simulink model "Monitor"  (R2022b)
settings: Solver=ode1  StartTime=0.0  StopTime=0.2  FixedStep=ctrlConst.TsSwitch  MaxStep=1e-6  RelTol=1e-3  EnableMultiTasking=on
PreLoadFcn:
  | %rtwdemo_pmsmfoc_data
StartFcn:
  | %clear executionProfile
StopFcn:
  | %try
  | %  AddExecutionProfileToDataInspector();
  | %end
undefined symbols (not defined in the file or in its folder): dataIphaOfsRawMon_C, facAdc2iPhMon_C, facAdc2uDclnkMon_C, KiRslvMonPI_C, KpRslvMonPI_C, Ld, Lq, Rss, SC_pMon_P, SC_PsiMon_P, tauTrqMonLv2_C, tauUdcPT1Mon_C, trqASCThdMonLv2_C, trqCmpThdMonLv2_C, Ts_10ms, Ts_1ms, Tsw
libraries: MathLib x14, IOLib x1, simulink x1
(part 2 of 2)

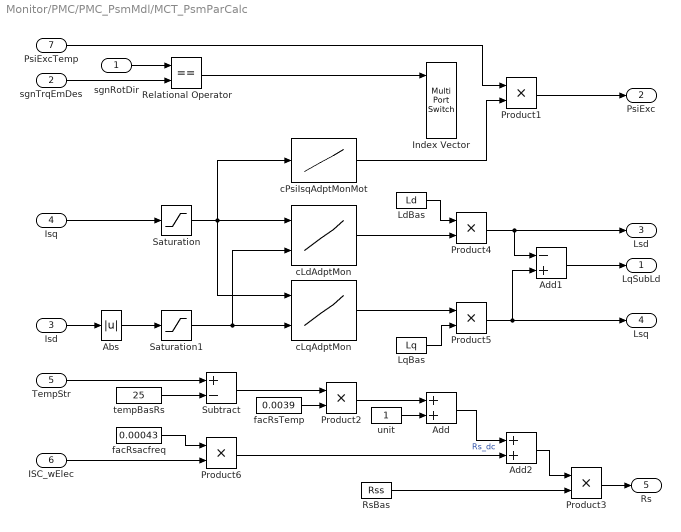
== system Monitor/PMC/PMC_PsmMdl/MCT_PsmParCalc ==
  sgnRotDir : Inport
  sgnTrqEmDes : Inport  Port=2
  Isd : Inport  Port=3
  Isq : Inport  Port=4
  TempStr : Inport  Port=5
  ISC_wElec : Inport  Port=6
  PsiExcTemp : Inport  Port=7
  Abs : Abs  SaturateOnIntegerOverflow=off
  Add : Sum  OutDataTypeStr=Inherit: Same as first input
  Add1 : Sum  Inputs=-+
  Add2 : Sum  OutDataTypeStr=Inherit: Same as first input
  Index Vector : MultiPortSwitch  DataPortOrder=Zero-based contiguous  Inputs=2  zeroidx=on  SaturateOnIntegerOverflow=off  InputSameDT=off
  LdBas : Constant  Value=Ld  OutDataTypeStr=single  SampleTime=-1
  LqBas : Constant  Value=Lq  OutDataTypeStr=single  SampleTime=-1
  Product1 : Product  OutDataTypeStr=single  RndMeth=Zero
  Product2 : Product  RndMeth=Zero
  Product3 : Product  RndMeth=Zero
  Product4 : Product  RndMeth=Zero  OutDataTypeStr=Inherit: Same as first input
  Product5 : Product  OutDataTypeStr=single  RndMeth=Zero
  Product6 : Product  RndMeth=Zero
  Relational Operator : RelationalOperator  Operator===  OutDataTypeStr=boolean  InputSameDT=off
  RsBas : Constant  Value=Rss  OutDataTypeStr=single  SampleTime=-1
  Saturation : Saturate  UpperLimit=450  LowerLimit=-450
  Saturation1 : Saturate  UpperLimit=450  LowerLimit=0
  Subtract : Sum  Inputs=+-
  cLdAdptMon : Lookup_n-D  DataSpecification=Lookup table object  LookupTableObject=cLdAdptMon_T  BreakpointsForDimension1=|  BreakpointsForDimension2=|  BeginIndexSearchUsingPreviousIndexResult=on  Table=|  ExtrapMethod=Clip  UseLastTableValue=on  InternalRulePriority=Speed  OutDataTypeStr=Inherit: Inherit from 'Table data'  InputSameDT=off
      BreakpointsForDimension1=|
      | [-530.4101839
      | -495.049505
      | -459.688826
      | -424.3281471
      | -388.9674682
      | -353.6067893
      | -318.2461103
      | -282.8854314
      | -247.5247525
      | -212.1640736
      | -176.8033946
      | -141.4427157
      | -106.0820368
      | -70.72135785
      | -35.36067893
      | 0
      | 35.36067893
      | 70.72135785
      | 106.0820368
      | 141.4427157
      | 176.8033946
      | 212.1640736
      | 247.5247525
      | 282.8854314
      | 318.2461103
      | 353.6067893
      | 388.9674682
      | 424.3281471
      | 459.688826
      | 495.049505
      | 530.4101839
      | ]
      BreakpointsForDimension2=|
      | [0	35.36067893	70.72135785	106.0820368	141.4427157	176.8033946	212.1640736	247.5247525	282.8854314	318.2461103	353.6067893	388.9674682	424.3281471	459.688826	495.049505	530.4101839
      | ]
      Table=|
      | [1	1	0.797297297	0.72972973	0.692567568	0.667567568	0.653153153	0.640926641	0.631756757	0.624624625	0.618918919	0.614742015	0.611486486	0.608731809	0.606177606	0.606177606
      | 1	1	0.797297297	0.72972973	0.692567568	0.667567568	0.653153153	0.640926641	0.631756757	0.624624625	0.618918919	0.614742015	0.611486486	0.608731809	0.606177606	0.606177606
      | 0.905405405	0.905405405	0.756756757	0.702702703	0.675675676	0.659459459	0.648648649	0.638996139	0.631756757	0.626126126	0.622972973	0.62002457	0.61768018	0.615800416	0.613899614	0.613899614
      | 0.810810811	0.810810811	0.716216216	0.68018018	0.665540541	0.651351351	0.644144144	0.638996139	0.633445946	0.630630631	0.628378378	0.626658477	0.625337838	0.624220374	0.622586873	0.622586873
      | 0.72972973	0.72972973	0.682432432	0.666666667	0.655405405	0.651351351	0.646396396	0.640926641	0.640202703	0.638138138	0.637027027	0.636240786	0.635585586	0.634927235	0.634169884	0.634169884
      | 0.635135135	0.635135135	0.648648649	0.648648649	0.648648649	0.648648649	0.646396396	0.646718147	0.64527027	0.645645646	0.646216216	0.646314496	0.646283784	0.646153846	0.645752896	0.645752896
      | 0.567567568	0.567567568	0.621621622	0.63963964	0.64527027	0.648648649	0.650900901	0.652509653	0.655405405	0.656606607	0.657837838	0.658562654	0.659009009	0.659043659	0.659266409	0.659266409
      | 0.513513514	0.513513514	0.601351351	0.630630631	0.64527027	0.654054054	0.65990991	0.664092664	0.665540541	0.67042042	0.672297297	0.673464373	0.674099099	0.674636175	0.673745174	0.673745174
      | 0.459459459	0.459459459	0.587837838	0.630630631	0.652027027	0.664864865	0.673423423	0.67953668	0.684121622	0.686786787	0.688918919	0.69017199	0.690653153	0.69022869	0.689189189	0.689189189
      | 0.432432432	0.432432432	0.587837838	0.63963964	0.668918919	0.683783784	0.695945946	0.702702703	0.706081081	0.709159159	0.710513514	0.713022113	0.710247748	0.708939709	0.707528958	0.707528958
      | 0.432432432	0.432432432	0.608108108	0.666666667	0.695945946	0.713513514	0.725225225	0.72972973	0.733108108	0.733483483	0.732986486	0.731572482	0.72972973	0.726611227	0.722972973	0.722972973
      | 0.486486486	0.486486486	0.662162162	0.716216216	0.743243243	0.754054054	0.761261261	0.760617761	0.760304054	0.758108108	0.755135135	0.751474201	0.747747748	0.742203742	0.737451737	0.737451737
      | 0.594594595	0.594594595	0.736486486	0.774774775	0.787162162	0.789189189	0.788288288	0.785714286	0.781756757	0.777027027	0.771891892	0.766093366	0.760135135	0.753638254	0.747104247	0.747104247
      | 0.72972973	0.72972973	0.804054054	0.81981982	0.820945946	0.818918919	0.813063063	0.806949807	0.8	0.792747748	0.78527027	0.777641278	0.77027027	0.761954262	0.754826255	0.754826255
      | 0.797297297	0.797297297	0.837837838	0.842342342	0.841216216	0.835135135	0.826576577	0.82046332	0.81097973	0.802012012	0.792837838	0.783783784	0.774774775	0.767151767	0.758687259	0.758687259
      | 0.790540541	0.790540541	0.834459459	0.84009009	0.837837838	0.832432432	0.82545045	0.818532819	0.809712838	0.800848348	0.791756757	0.782555283	0.774211712	0.766112266	0.757722008	0.757722008
      | 0.783783784	0.783783784	0.831081081	0.837837838	0.834459459	0.82972973	0.824324324	0.816602317	0.808445946	0.799684685	0.790675676	0.781326781	0.773648649	0.765072765	0.756756757	0.756756757
      | 0.689189189	0.689189189	0.783783784	0.806306306	0.810810811	0.810810811	0.806306306	0.801158301	0.794932432	0.788243243	0.781216216	0.773710074	0.765765766	0.758835759	0.751930502	0.751930502
      | 0.554054054	0.554054054	0.716216216	0.756756757	0.773648649	0.781081081	0.781531532	0.77992278	0.776013514	0.771921922	0.767162162	0.761793612	0.755630631	0.749480249	0.744208494	0.744208494
      | 0.418918919	0.418918919	0.628378378	0.693693694	0.726351351	0.743243243	0.75	0.752895753	0.752195946	0.750900901	0.748513514	0.745331695	0.742117117	0.737006237	0.732625483	0.732625483
      | 0.351351351	0.351351351	0.567567568	0.63963964	0.675675676	0.697297297	0.709459459	0.718146718	0.722972973	0.724024024	0.736459459	0.723587224	0.721846847	0.719334719	0.716216216	0.716216216
      | 0.351351351	0.351351351	0.547297297	0.612612613	0.64527027	0.664864865	0.677927928	0.687258687	0.694256757	0.697747748	0.7	0.701105651	0.701238739	0.700623701	0.698841699	0.698841699
      | 0.378378378	0.378378378	0.547297297	0.599099099	0.628378378	0.662162162	0.657657658	0.666023166	0.670608108	0.675375375	0.678378378	0.68034398	0.681418919	0.681912682	0.681467181	0.681467181
      | 0.405405405	0.405405405	0.547297297	0.594594595	0.618243243	0.632432432	0.641891892	0.646718147	0.652027027	0.656306306	0.659189189	0.661277641	0.662725225	0.663201663	0.664092664	0.664092664
      | 0.459459459	0.459459459	0.560810811	0.599099099	0.614864865	0.624324324	0.630630631	0.635135135	0.638513514	0.641141141	0.643648649	0.64546683	0.646734234	0.647609148	0.647683398	0.647683398
      | 0.513513514	0.513513514	0.587837838	0.608108108	0.614864865	0.618918919	0.623873874	0.625482625	0.628378378	0.629129129	0.631216216	0.632309582	0.633220721	0.633783784	0.634169884	0.634169884
      | 0.594594595	0.594594595	0.614864865	0.621621622	0.621621622	0.621621622	0.619369369	0.61969112	0.619932432	0.62012012	0.621081081	0.621498771	0.621734234	0.621933472	0.621621622	0.621621622
      | 0.675675676	0.675675676	0.641891892	0.635135135	0.628378378	0.624324324	0.619369369	0.617760618	0.614864865	0.614114114	0.612837838	0.612285012	0.611936937	0.611538462	0.611003861	0.611003861
      | 0.756756757	0.756756757	0.682432432	0.653153153	0.638513514	0.62972973	0.621621622	0.615830116	0.611486486	0.608108108	0.606351351	0.604545455	0.603502252	0.602494802	0.601640927	0.601640927
      | 0.851351351	0.851351351	0.716216216	0.675675676	0.652027027	0.635135135	0.623873874	0.615830116	0.609797297	0.605105105	0.601216216	0.598525799	0.596418919	0.594698545	0.593243243	0.593243243
      | 0.851351351	0.851351351	0.716216216	0.675675676	0.652027027	0.635135135	0.623873874	0.615830116	0.609797297	0.605105105	0.601216216	0.598525799	0.596418919	0.594698545	0.593243243	0.593243243
      | ]
      settings: InputPortMap=u0,u1
  cLqAdptMon : Lookup_n-D  DataSpecification=Lookup table object  LookupTableObject=cLqAdptMon_T  BreakpointsForDimension1=|  BreakpointsForDimension2=|  BeginIndexSearchUsingPreviousIndexResult=on  Table=|  ExtrapMethod=Clip  UseLastTableValue=on  InternalRulePriority=Speed  OutDataTypeStr=Inherit: Inherit from 'Table data'  InputSameDT=off
      BreakpointsForDimension1=|
      | [-530.4101839
      | -495.049505
      | -459.688826
      | -424.3281471
      | -388.9674682
      | -353.6067893
      | -318.2461103
      | -282.8854314
      | -247.5247525
      | -212.1640736
      | -176.8033946
      | -141.4427157
      | -106.0820368
      | -70.72135785
      | -35.36067893
      | 0
      | 35.36067893
      | 70.72135785
      | 106.0820368
      | 141.4427157
      | 176.8033946
      | 212.1640736
      | 247.5247525
      | 282.8854314
      | 318.2461103
      | 353.6067893
      | 388.9674682
      | 424.3281471
      | 459.688826
      | 495.049505
      | 530.4101839
      | ]
      BreakpointsForDimension2=|
      | [0	35.36067893	70.72135785	106.0820368	141.4427157	176.8033946	212.1640736	247.5247525	282.8854314	318.2461103	353.6067893	388.9674682	424.3281471	459.688826	495.049505	530.4101839
      | ]
      Table=|
      | [0.394500897	0.39748954	0.39748954	0.400478183	0.403466826	0.403466826	0.403466826	0.406455469	0.406455469	0.406455469	0.403466826	0.403466826	0.403466826	0.400478183	0.400478183	0.400478183
      | 0.394500897	0.39748954	0.39748954	0.400478183	0.403466826	0.403466826	0.403466826	0.406455469	0.406455469	0.406455469	0.403466826	0.403466826	0.403466826	0.400478183	0.400478183	0.400478183
      | 0.418410042	0.421628581	0.424847119	0.424847119	0.428065658	0.428065658	0.428065658	0.428065658	0.431284197	0.428065658	0.428065658	0.428065658	0.424847119	0.424847119	0.421628581	0.421628581
      | 0.446304045	0.449790795	0.453277545	0.453277545	0.456764296	0.456764296	0.456764296	0.456764296	0.456764296	0.456764296	0.453277545	0.453277545	0.449790795	0.449790795	0.446304045	0.446304045
      | 0.479269684	0.483073412	0.483073412	0.48687714	0.48687714	0.48687714	0.48687714	0.48687714	0.48687714	0.48687714	0.483073412	0.483073412	0.479269684	0.475465957	0.471662229	0.471662229
      | 0.514644351	0.518828452	0.518828452	0.523012552	0.523012552	0.523012552	0.523012552	0.523012552	0.523012552	0.518828452	0.514644351	0.514644351	0.510460251	0.506276151	0.49790795	0.49790795
      | 0.557880056	0.562529056	0.562529056	0.562529056	0.562529056	0.562529056	0.562529056	0.562529056	0.557880056	0.557880056	0.553231055	0.548582055	0.543933054	0.534635053	0.529986053	0.529986053
      | 0.606694561	0.611924686	0.611924686	0.611924686	0.611924686	0.611924686	0.606694561	0.606694561	0.601464435	0.59623431	0.591004184	0.585774059	0.575313808	0.570083682	0.559623431	0.559623431
      | 0.669456067	0.669456067	0.669456067	0.669456067	0.669456067	0.663478781	0.663478781	0.657501494	0.651524208	0.639569635	0.633592349	0.621637776	0.61566049	0.603705918	0.593544531	0.593544531
      | 0.739191074	0.739191074	0.739191074	0.732217573	0.732217573	0.725244073	0.718270572	0.711297071	0.69735007	0.686889819	0.675034868	0.663179916	0.650627615	0.637377964	0.624825662	0.624825662
      | 0.816736402	0.815899582	0.812552301	0.806694561	0.79748954	0.785774059	0.772384937	0.758158996	0.743933054	0.728870293	0.713807531	0.69790795	0.682845188	0.667782427	0.652719665	0.652719665
      | 0.900627615	0.894351464	0.882845188	0.868200837	0.851464435	0.833682008	0.815899582	0.79707113	0.779288703	0.761506276	0.743723849	0.725941423	0.708158996	0.691422594	0.675732218	0.675732218
      | 0.965132497	0.949790795	0.928870293	0.907949791	0.885634589	0.864714086	0.845188285	0.824267782	0.80334728	0.782426778	0.762900976	0.741980474	0.723849372	0.705718271	0.688981869	0.688981869
      | 0.991631799	0.972803347	0.951882845	0.930962343	0.907949791	0.887029289	0.864016736	0.838912134	0.815899582	0.728033473	0.769874477	0.748953975	0.728033473	0.709205021	0.690376569	0.690376569
      | 1	0.979079498	0.958158996	0.937238494	0.920502092	0.89539749	0.866108787	0.841004184	0.811715481	0.786610879	0.757322176	0.736401674	0.715481172	0.690376569	0.673640167	0.673640167
      | 1	0.981171548	0.964435146	0.947698745	0.933054393	0.910041841	0.884937238	0.861924686	0.836820084	0.813807531	0.790794979	0.771966527	0.755230126	0.734309623	0.719665272	0.719665272
      | 1	0.983263598	0.970711297	0.958158996	0.945606695	0.924686192	0.90376569	0.882845188	0.861924686	0.841004184	0.824267782	0.807531381	0.794979079	0.778242678	0.765690377	0.765690377
      | 0.991631799	0.951882845	0.958158996	0.939330544	0.920502092	0.90167364	0.882845188	0.861924686	0.841004184	0.820083682	0.80125523	0.784518828	0.767782427	0.751046025	0.738493724	0.738493724
      | 0.965132497	0.951185495	0.933054393	0.913528591	0.894002789	0.875871688	0.857740586	0.839609484	0.820083682	0.80195258	0.783821478	0.767085077	0.750348675	0.735006974	0.719665272	0.719665272
      | 0.900627615	0.896443515	0.887029289	0.873430962	0.857740586	0.842050209	0.825313808	0.808577406	0.791841004	0.776150628	0.759414226	0.743723849	0.728033473	0.712343096	0.697698745	0.697698745
      | 0.816736402	0.817573222	0.815062762	0.810041841	0.80167364	0.791631799	0.779916318	0.767364017	0.753974895	0.739748954	0.725523013	0.711297071	0.69790795	0.683682008	0.670292887	0.670292887
      | 0.739191074	0.739191074	0.739191074	0.739191074	0.732217573	0.732217573	0.725244073	0.711297071	0.70432357	0.69525802	0.684797768	0.673640167	0.661785216	0.649930265	0.638075314	0.638075314
      | 0.669456067	0.669456067	0.669456067	0.669456067	0.669456067	0.669456067	0.663478781	0.657501494	0.657501494	0.645546922	0.639569635	0.633592349	0.621637776	0.61566049	0.603705918	0.603705918
      | 0.606694561	0.611924686	0.611924686	0.611924686	0.611924686	0.611924686	0.611924686	0.611924686	0.606694561	0.601464435	0.59623431	0.591004184	0.585774059	0.575313808	0.570083682	0.570083682
      | 0.557880056	0.562529056	0.562529056	0.567178057	0.567178057	0.567178057	0.567178057	0.562529056	0.562529056	0.557880056	0.557880056	0.553231055	0.548582055	0.543933054	0.539284054	0.539284054
      | 0.514644351	0.518828452	0.518828452	0.523012552	0.523012552	0.527196653	0.527196653	0.527196653	0.523012552	0.523012552	0.518828452	0.518828452	0.514644351	0.510460251	0.506276151	0.506276151
      | 0.479269684	0.479269684	0.483073412	0.48687714	0.48687714	0.490680867	0.490680867	0.490680867	0.490680867	0.490680867	0.48687714	0.48687714	0.483073412	0.479269684	0.475465957	0.475465957
      | 0.446304045	0.449790795	0.453277545	0.453277545	0.456764296	0.456764296	0.456764296	0.460251046	0.460251046	0.460251046	0.456764296	0.456764296	0.453277545	0.453277545	0.449790795	0.449790795
      | 0.418410042	0.421628581	0.424847119	0.424847119	0.428065658	0.428065658	0.431284197	0.431284197	0.431284197	0.431284197	0.431284197	0.431284197	0.428065658	0.428065658	0.424847119	0.424847119
      | 0.394500897	0.39748954	0.39748954	0.400478183	0.403466826	0.403466826	0.406455469	0.406455469	0.406455469	0.406455469	0.406455469	0.406455469	0.406455469	0.403466826	0.403466826	0.403466826
      | 0.394500897	0.39748954	0.39748954	0.400478183	0.403466826	0.403466826	0.406455469	0.406455469	0.406455469	0.406455469	0.406455469	0.406455469	0.406455469	0.403466826	0.403466826	0.403466826
      | ]
      settings: InputPortMap=u0,u1
  cPsiIsqAdptMonMot : Lookup_n-D  NumberOfTableDimensions=1  DataSpecification=Lookup table object  LookupTableObject=cPsiIsqAdptMonMot_T  BreakpointsForDimension1=|  BeginIndexSearchUsingPreviousIndexResult=on  Table=|  ExtrapMethod=Clip  UseLastTableValue=on  InternalRulePriority=Speed  OutDataTypeStr=Inherit: Inherit from 'Table data'
      BreakpointsForDimension1=|
      | [-530.4101839
      | -495.049505
      | -459.688826
      | -424.3281471
      | -388.9674682
      | -353.6067893
      | -318.2461103
      | -282.8854314
      | -247.5247525
      | -212.1640736
      | -176.8033946
      | -141.4427157
      | -106.0820368
      | -70.72135785
      | -35.36067893
      | 0
      | 35.36067893
      | 70.72135785
      | 106.0820368
      | 141.4427157
      | 176.8033946
      | 212.1640736
      | 247.5247525
      | 282.8854314
      | 318.2461103
      | 353.6067893
      | 388.9674682
      | 424.3281471
      | 459.688826
      | 495.049505
      | 530.4101839
      | ]
      Table=|
      | [0.983333333
      | 0.983333333
      | 0.985185185
      | 0.987037037
      | 0.990740741
      | 0.992592593
      | 0.994444444
      | 0.996296296
      | 0.996296296
      | 0.998148148
      | 0.998148148
      | 0.998148148
      | 0.994444444
      | 0.992592593
      | 0.990740741
      | 0.990740741
      | 0.990740741
      | 0.992592593
      | 0.996296296
      | 1
      | 1
      | 1
      | 1
      | 0.998148148
      | 0.996296296
      | 0.994444444
      | 0.992592593
      | 0.990740741
      | 0.988888889
      | 0.987037037
      | 0.987037037]
  facRsTemp : Constant  Value=0.0039  OutDataTypeStr=single  SampleTime=-1
  facRsacfreq : Constant  Value=0.00043  OutDataTypeStr=single  SampleTime=-1
  tempBasRs : Constant  Value=25  OutDataTypeStr=single  SampleTime=-1
  unit : Constant  OutDataTypeStr=single  SampleTime=-1
  LqSubLd : Outport  VectorParamsAs1DForOutWhenUnconnected=off
  PsiExc : Outport  Port=2  VectorParamsAs1DForOutWhenUnconnected=off
  Lsd : Outport  Port=3  VectorParamsAs1DForOutWhenUnconnected=off
  Lsq : Outport  Port=4  VectorParamsAs1DForOutWhenUnconnected=off
  Rs : Outport  Port=5  VectorParamsAs1DForOutWhenUnconnected=off
  wires:
  PsiExcTemp/1 -> Product1/1
  Add1/1 -> LqSubLd/1
  Product5/1 -> Add1/2, Lsq/1
  Product4/1 -> Add1/1, Lsd/1
  Product1/1 -> PsiExc/1
  Product3/1 -> Rs/1
  LqBas/1 -> Product5/2
  cLqAdptMon/1 -> Product5/1
  cLdAdptMon/1 -> Product4/2
  LdBas/1 -> Product4/1
  Abs/1 -> Saturation1/1
  Isq/1 -> Saturation/1
  RsBas/1 -> Product3/2
  Add/1 -> Add2/1  "Rs_dc"
  unit/1 -> Add/2
  Product2/1 -> Add/1
  facRsTemp/1 -> Product2/2
  Subtract/1 -> Product2/1
  tempBasRs/1 -> Subtract/2
  TempStr/1 -> Subtract/1
  Isd/1 -> Abs/1
  Relational Operator/1 -> Index Vector/1
  sgnTrqEmDes/1 -> Relational Operator/2
  sgnRotDir/1 -> Relational Operator/1
  cPsiIsqAdptMonMot/1 -> Product1/2
  ISC_wElec/1 -> Product6/2
  Product6/1 -> Add2/2
  Add2/1 -> Product3/1
  facRsacfreq/1 -> Product6/1
  Saturation/1 -> cLqAdptMon/1, cLdAdptMon/1, cPsiIsqAdptMonMot/1
  Saturation1/1 -> cLqAdptMon/2, cLdAdptMon/2

== matlab function Monitor/TCP/trigerLock ==
  data: out output; trigger input
function out = fcn(trigger)
%
persistent outTmp;

if isempty(outTmp)
    outTmp = false;
end

if trigger
    outTmp = true;
end

out = outTmp;

== matlab function Monitor/ISP/ISP_Ana/ISP_AnaCalnPosCalnMon/Position PI Observer ==
  data: frqCal input; dAngle input; freq output; tiPerd input; Comp1 output; Comp2 output; Ki input; Kp input
function [freq, Comp1, Comp2]   = fcn(frqCal, dAngle, tiPerd, Ki, Kp)
%Debug record
%
%
persistent dIntFreq;
persistent ActFreq;
persistent cntRstRslv;
persistent flgObsrRslv;

if isempty(dIntFreq)
    dIntFreq = single(0);
    ActFreq = single(0);
    cntRstRslv = uint8(0);
    flgObsrRslv = false;
end

MaxFreq = single(2000);

if flgObsrRslv==true 
    dKp = Kp * dAngle;
    dKi = Ki * dAngle; 

    dIntFreq=dIntFreq+dKi;

    if dIntFreq > MaxFreq
       dIntFreq = MaxFreq;
    else
        if dIntFreq < (-MaxFreq)
            dIntFreq = (-MaxFreq);
        end
    end

    freq = dKp + dIntFreq;

    if freq > MaxFreq
       freq = MaxFreq;
    else
        if freq < (-MaxFreq)
            freq = (-MaxFreq);
        end
    end
else
    cntRstRslv = cntRstRslv + uint8(1);

    if cntRstRslv>uint8(100)
        flgObsrRslv = true;
        dIntFreq = frqCal;
    end
    
    freq = frqCal;
end

ActFreq = freq;

%compensation
Comp1 = ActFreq*single(0.065535)*tiPerd;

%compensation
Comp2 = ActFreq*single(0.032767)*tiPerd;

== matlab function Monitor/ISP/ISP_Ana/ISP_AnaCalnIpha/MaxMinValueCal ==
  data: ipha1 input; ipha2 input; dataIpha1MaxOut output; dataIpha1MinOut output; ipha3 input; dataIpha2MaxOut output; dataIpha2MinOut output; dataIpha3MaxOut output; dataIpha3MinOut output
function [dataIpha1MaxOut,dataIpha1MinOut,dataIpha2MaxOut,dataIpha2MinOut,dataIpha3MaxOut,dataIpha3MinOut]   = fcn(ipha1,ipha2,ipha3)
%Debug record
%
%
persistent cntrIphaMaxCal;
persistent dataIpha1Max;
persistent dataIpha1Min;
persistent dataIpha2Max;
persistent dataIpha2Min;
persistent dataIpha3Max;
persistent dataIpha3Min;
persistent ipha1MaxCal;
persistent ipha1MinCal;
persistent ipha2MaxCal;
persistent ipha2MinCal;
persistent ipha3MaxCal;
persistent ipha3MinCal;

if isempty(cntrIphaMaxCal)
    cntrIphaMaxCal = uint8(0);
    dataIpha1Max = uint16(32767);
    dataIpha1Min = uint16(32767);
    dataIpha2Max = uint16(32767);
    dataIpha2Min = uint16(32767);
    dataIpha3Max = uint16(32767);
    dataIpha3Min = uint16(32767);
    ipha1MaxCal = uint16(32767);
    ipha1MinCal = uint16(32767);
    ipha2MaxCal = uint16(32767);
    ipha2MinCal = uint16(32767);
    ipha3MaxCal = uint16(32767);
    ipha3MinCal = uint16(32767);
end

if cntrIphaMaxCal>uint8(9)
    cntrIphaMaxCal = uint8(0);
    
    if ipha1> dataIpha1Max
        ipha1MaxCal =  ipha1;
    else
        ipha1MaxCal = dataIpha1Max;
    end
    
    if ipha1<dataIpha1Min
        ipha1MinCal = ipha1;
    else
        ipha1MinCal = dataIpha1Min;
    end
    
    if ipha2> dataIpha2Max
        ipha2MaxCal =  ipha2;
    else
        ipha2MaxCal = dataIpha2Max;
    end
    
    if ipha2<dataIpha2Min
        ipha2MinCal = ipha2;
    else
        ipha2MinCal = dataIpha2Min;
    end
    
    if ipha3> dataIpha3Max
        ipha3MaxCal =  ipha3;
    else
        ipha3MaxCal = dataIpha3Max;
    end
    
    if ipha3<dataIpha3Min
        ipha3MinCal = ipha3;
    else
        ipha3MinCal = dataIpha3Min;
    end
    
    dataIpha1Max = uint16(32767);
    dataIpha1Min = uint16(32767);
    dataIpha2Max = uint16(32767);
    dataIpha2Min = uint16(32767);
    dataIpha3Max = uint16(32767);
    dataIpha3Min = uint16(32767);
else
    cntrIphaMaxCal = cntrIphaMaxCal + uint8(1);
    
    if ipha1> dataIpha1Max
        dataIpha1Max =  ipha1;
    end
    
    if ipha1<dataIpha1Min
        dataIpha1Min = ipha1;
    end
    
    if ipha2> dataIpha2Max
        dataIpha2Max =  ipha2;
    end
    
    if ipha2<dataIpha2Min
        dataIpha2Min = ipha2;
    end
   
    if ipha3> dataIpha3Max
        dataIpha3Max =  ipha3;
    end
    
    if ipha3<dataIpha3Min
        dataIpha3Min = ipha3;
    end
end

dataIpha1MaxOut = ipha1MaxCal;
dataIpha1MinOut = ipha1MinCal;
dataIpha2MaxOut = ipha2MaxCal;
dataIpha2MinOut = ipha2MinCal;
dataIpha3MaxOut = ipha3MaxCal;
dataIpha3MinOut = ipha3MinCal;
